simulink model "skok"  (R2017b)
settings: Solver=VariableStepAuto  StartTime=0.0  StopTime=20  RelTol=1e-3
values from neighbouring files (symbols this model uses):
  ki = [0 1 15]    [lab2_skok.m]
  kp = [1 7 15]    [lab2_skok.m]
  M = [[0 0 1 1]; [1 3 3 1]]    [lab2_skok.m]
undefined symbols (not defined in the file or in its folder): g, i, s
settings Model: Creator=Witaj Przemku  LastModifiedBy=lev
settings CodeAppCC: StateflowObjectComments=on

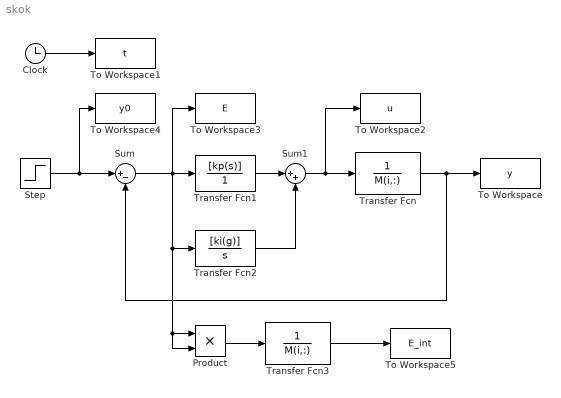
== system skok ==
  Clock : Clock
  Product : Product
  Step : Step  Time=0  SampleTime=0
  Sum : Sum  Inputs=|+-
  Sum1 : Sum  Inputs=|++
  To Workspace : ToWorkspace  VariableName=y  SampleTime=0.1
      settings: Save2DSignal=2-D array (concatenate along first dimension)
  To Workspace1 : ToWorkspace  VariableName=t  SampleTime=0.1
      settings: Save2DSignal=2-D array (concatenate along first dimension)
  To Workspace2 : ToWorkspace  VariableName=u  SampleTime=0.1
      settings: Save2DSignal=2-D array (concatenate along first dimension)
  To Workspace3 : ToWorkspace  VariableName=E  SampleTime=0.1
      settings: Save2DSignal=2-D array (concatenate along first dimension)
  To Workspace4 : ToWorkspace  VariableName=y0  SampleTime=0.1
      settings: Save2DSignal=2-D array (concatenate along first dimension)
  To Workspace5 : ToWorkspace  VariableName=E_int  SampleTime=0.1
      settings: Save2DSignal=2-D array (concatenate along first dimension)
  Transfer Fcn : TransferFcn  Denominator=M(i,:)
  Transfer Fcn1 : TransferFcn  Numerator=[kp(s)]  Denominator=[1]
  Transfer Fcn2 : TransferFcn  Numerator=[ki(g)]  Denominator=[1 0]
  Transfer Fcn3 : TransferFcn  Denominator=M(i,:)
  wires:
  Clock/1 -> To Workspace1/1
  Sum/1 -> Product/2, Product/1, Transfer Fcn2/1, Transfer Fcn1/1, To Workspace3/1
  Step/1 -> To Workspace4/1, Sum/1
  Transfer Fcn/1 -> Sum/2, To Workspace/1
  Sum1/1 -> To Workspace2/1, Transfer Fcn/1
  Transfer Fcn1/1 -> Sum1/1
  Transfer Fcn2/1 -> Sum1/2
  Product/1 -> Transfer Fcn3/1
  Transfer Fcn3/1 -> To Workspace5/1
